simulink model "MotorDCmodel"  (R2014a)
settings: Solver=ode45  StartTime=0.0  StopTime=100  RelTol=1e-2
values from neighbouring files (symbols this model uses):
  B = Bi    (= 0.0025)    [MotorDC.m]
  J = Ji    (= 0.0015)    [MotorDC.m]
  Ke = 0.021 *60/w    (= 0.00334225380493)    [MotorDC.m]
  Kt = 0.2    [MotorDC.m]
  L = 3e-5    (= 3e-05)    [MotorDC.m]
  R = 8    [MotorDC.m]
libraries: simulink x1
settings Model: Creator=Eduardo  LastModifiedBy=Eduardo

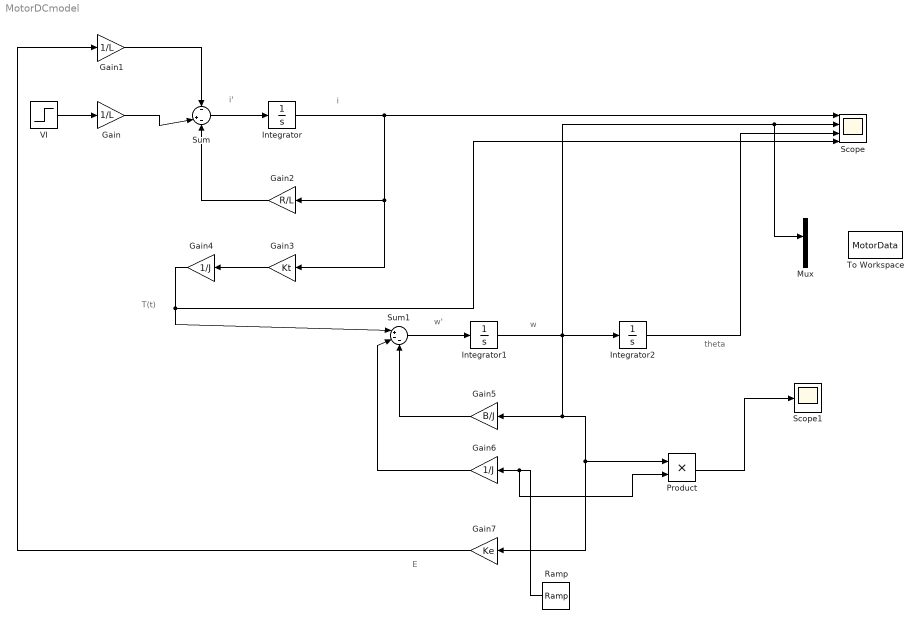
== system MotorDCmodel ==
  note: E
  note: theta
  note: w
  note: w'
  note: T(t)
  note: i
  note: i'
  Gain : Gain  Gain=1/L
  Gain1 : Gain  Gain=1/L
  Gain2 : Gain  Gain=R/L
  Gain3 : Gain  Gain=Kt
  Gain4 : Gain  Gain=1/J
  Gain5 : Gain  Gain=B/J
  Gain6 : Gain  Gain=1/J
  Gain7 : Gain  Gain=Ke
  Integrator : Integrator
  Integrator1 : Integrator
  Integrator2 : Integrator
  Mux : Mux
  Product : Product
  Ramp : simulink/Sources/Ramp  slope=0.6  start=100  X0=0
  Scope : Scope  NumInputPorts=4
      settings: TimeRange=6  YMin=-5~-5~-5~-5  YMax=5~5~5~5
  Scope1 : Scope
  Sum : Sum  Inputs=-|+-
  Sum1 : Sum  Inputs=|+--
  To Workspace : ToWorkspace  VariableName=MotorData  SaveFormat=Timeseries  SampleTime=-1
  VI : Step  After=20  SampleTime=0
  wires:
  VI/1 -> Gain/1
  Sum/1 -> Integrator/1
  Integrator/1 -> Scope/1, Gain3/1, Gain2/1
  Gain/1 -> Sum/2
  Gain1/1 -> Sum/1
  Gain2/1 -> Sum/3
  Gain3/1 -> Gain4/1
  Sum1/1 -> Integrator1/1
  Integrator1/1 -> Gain5/1, Product/1, Gain7/1, Mux/2, Scope/2, Integrator2/1
  Gain4/1 -> Scope/4, Sum1/1
  Gain5/1 -> Sum1/3
  Ramp/1 -> Product/2, Gain6/1
  Gain6/1 -> Sum1/2
  Integrator2/1 -> Scope/3
  Gain7/1 -> Gain1/1
  Product/1 -> Scope1/1
